simulink model "bloque_fil"  (R2017a)
settings: Solver=VariableStepAuto  StartTime=0.0  StopTime=0.01  FixedStep=0.595e-6  RelTol=1e-3
libraries: fillib x1
settings Model: Creator=Javier  LastModifiedBy=Javier

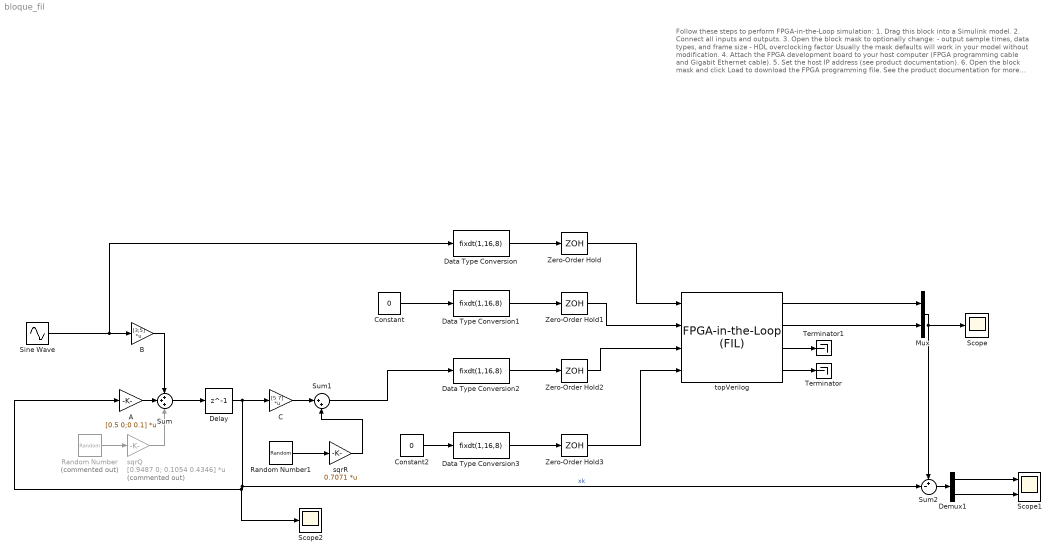
== system bloque_fil ==
  note: Follow these steps to perform FPGA-in-the-Loop simulation:
      |
      | 1. Drag this block into a Simulink model.
      | 2. Connect all inputs and outputs.
      | 3. Open the block mask to optionally change:
      |     - output sample times, data types, and frame size
      |     - HDL overclocking factor
      |     Usually the mask defaults will work in your model without modification.
      | 4. Attach the FPGA development board to your host computer (FPGA
      |     programming cable and Gigabit Ethernet cable).
      | 5. Set the host IP address (see product documentation).
      | 6. Open the block mask and click Load to download the FPGA programming file.
      |
      | See the product documentation for more detailed instructions and
      | troubleshooting tips.
  A : Gain  Gain=[0.5 0;0 0.1]  Multiplication=Matrix(K*u) (u vector)
  B : Gain  Gain=[3;5]  Multiplication=Matrix(K*u)
  C : Gain  Gain=[5 7]  Multiplication=Matrix(K*u)
  Constant : Constant  Value=0
  Constant2 : Constant  Value=0
  Data Type Conversion{,1..3} (4 alike) : DataTypeConversion  OutDataTypeStr=fixdt(1,16,8)  SaturateOnIntegerOverflow=on
  Delay : Delay  DelayLength=1  InitialCondition=0  SampleTime=1.19e-6
  Demux1 : Demux  Outputs=2
  Mux : Mux  Inputs=2
  Random Number : RandomNumber  Commented=on  Variance=[1; 1]  SampleTime=1.19e-6
  Random Number1 : RandomNumber  SampleTime=1.19e-6
  Scope : Scope
  Scope1 : Scope  NumInputPorts=2
  Scope2 : Scope
  Sine Wave : Sin  Frequency=2*pi*100  SampleTime=1.19e-6
  Sum : Sum  Inputs=+++
  Sum1 : Sum  Inputs=|++
  Sum2 : Sum  Inputs=+-|
  Terminator : Terminator
  Terminator1 : Terminator
  Zero-Order Hold{,1..3} (4 alike) : ZeroOrderHold  SampleTime=1.19e-6
  sqrQ : Gain  Commented=on  Gain=[0.9487 0; 0.1054 0.4346]  Multiplication=Matrix(K*u)
  sqrR : Gain  Gain=0.7071  Multiplication=Matrix(K*u)
  topVerilog : fillib/FPGA-in-the-Loop (FIL)  ForceInterfaceUpdate=0.81472
  wires:
  Data Type Conversion/1 -> Zero-Order Hold/1
  Data Type Conversion1/1 -> Zero-Order Hold1/1
  Data Type Conversion2/1 -> Zero-Order Hold2/1
  Data Type Conversion3/1 -> Zero-Order Hold3/1
  Constant/1 -> Data Type Conversion1/1
  Zero-Order Hold1/1 -> topVerilog/2
  Zero-Order Hold/1 -> topVerilog/1
  Zero-Order Hold2/1 -> topVerilog/3
  Zero-Order Hold3/1 -> topVerilog/4
  topVerilog/4 -> Terminator/1
  Mux/1 -> Sum2/1, Scope/1
  topVerilog/1 -> Mux/1
  topVerilog/2 -> Mux/2
  Sine Wave/1 -> Data Type Conversion/1, B/1
  A/1 -> Sum/2
  Sum/1 -> Delay/1
  Delay/1 -> Scope2/1, A/1, Sum2/2, C/1  "xk"
  B/1 -> Sum/1
  Sum1/1 -> Data Type Conversion2/1
  Random Number/1 -> sqrQ/1
  sqrQ/1 -> Sum/3
  Random Number1/1 -> sqrR/1
  Sum2/1 -> Demux1/1
  Demux1/1 -> Scope1/1
  Demux1/2 -> Scope1/2
  topVerilog/3 -> Terminator1/1
  Constant2/1 -> Data Type Conversion3/1
  sqrR/1 -> Sum1/2
  C/1 -> Sum1/1
